simulink model "Motor_Step_Response_Linear_1st_2nd_Coulomb"  (R2016b)
settings: Solver=ode5  StartTime=0.0  StopTime=Tsim_final  FixedStep=sim_step_size  RelTol=1e-3
values from neighbouring files (symbols this model uses):
  Bm = 0    [HW6pt2.m]    (also in Homework_5_Justin_Garcia.m; Motor_Parameters.m = 0.01; Motor_Parameters_2.m = 0.01)
  Jm = .002    (= 0.002)    [Motor_Parameters.m]    (also in Motor_Parameters_2.m)
  Kb = .7    (= 0.7)    [Motor_Parameters.m]    (also in Motor_Parameters_2.m)
  Kt = .7    (= 0.7)    [Motor_Parameters.m]    (also in Motor_Parameters_2.m)
  Lm = .004    (= 0.004)    [Motor_Parameters.m]    (also in Motor_Parameters_2.m)
  Rm = 10    [Motor_Parameters.m]    (also in Motor_Parameters_2.m)
  Tf = 0    [HW6pt2.m]    (also in Homework_5_Justin_Garcia.m; Motor_Parameters.m = 0.02; Motor_Parameters_2.m = 0.02)
  Vsupply = 4.5    [Motor_Parameters.m]    (also in Motor_Parameters_2.m)
settings Model: Creator=Mac  LastModifiedBy=Mac

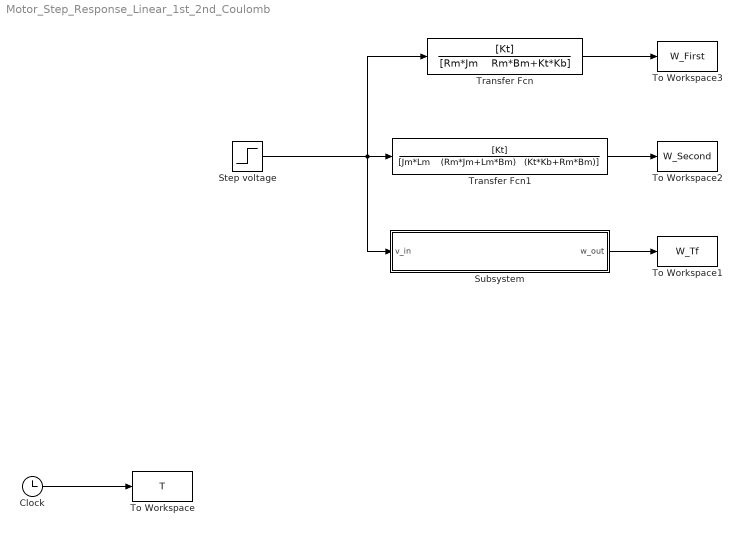
== system Motor_Step_Response_Linear_1st_2nd_Coulomb ==
  Clock : Clock
  Step voltage : Step  Time=0  After=Vsupply  SampleTime=0
  Subsystem : Subsystem
  To Workspace : ToWorkspace  VariableName=T  SampleTime=-1
  To Workspace1 : ToWorkspace  VariableName=W_Tf  SampleTime=-1
  To Workspace2 : ToWorkspace  VariableName=W_Second  SampleTime=-1
  To Workspace3 : ToWorkspace  VariableName=W_First  SampleTime=-1
  Transfer Fcn : TransferFcn  Numerator=[Kt]  Denominator="[Rm*Jm    Rm*Bm+Kt*Kb]"
  Transfer Fcn1 : TransferFcn  Numerator=[Kt]  Denominator="[Jm*Lm    (Rm*Jm+Lm*Bm)   (Kt*Kb+Rm*Bm)]"
  wires:
  Clock/1 -> To Workspace/1
  Transfer Fcn/1 -> To Workspace3/1
  Transfer Fcn1/1 -> To Workspace2/1
  Subsystem/1(w_out) -> To Workspace1/1
  Step voltage/1 -> Subsystem/1(v_in), Transfer Fcn1/1, Transfer Fcn/1

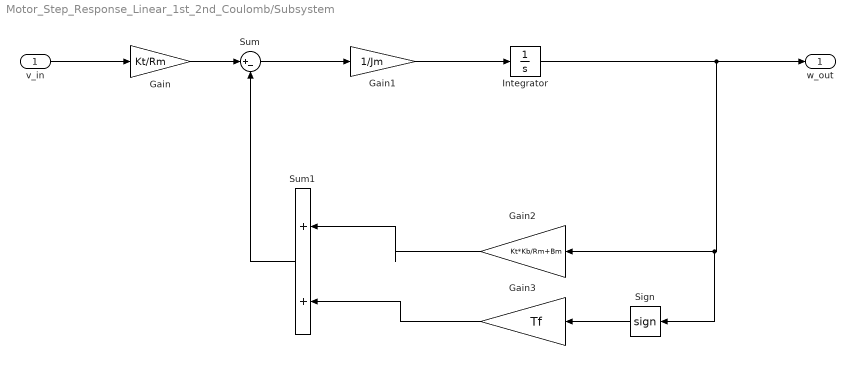
== system Motor_Step_Response_Linear_1st_2nd_Coulomb/Subsystem ==
  v_in : Inport
  Gain : Gain  Gain=Kt/Rm
  Gain1 : Gain  Gain=1/Jm
  Gain2 : Gain  Gain=Kt*Kb/Rm+Bm
  Gain3 : Gain  Gain=Tf
  Integrator : Integrator
  Sign : Signum
  Sum : Sum  Inputs=|+-
  Sum1 : Sum  Inputs=|++
  w_out : Outport
  wires:
  Integrator/1 -> Sign/1, Gain2/1, w_out/1
  Gain1/1 -> Integrator/1
  Sum/1 -> Gain1/1
  Gain/1 -> Sum/1
  Sum1/1 -> Sum/2
  Gain2/1 -> Sum1/1
  Gain3/1 -> Sum1/2
  Sign/1 -> Gain3/1
  v_in/1 -> Gain/1
